simulink model "ProblemaTanques20240610"  (R2023b)
settings: Solver=ode4  StartTime=0.0  StopTime=100  FixedStep=.001  RelTol=1e-3
values from neighbouring files (symbols this model uses):
  Ts = 0.005    [Problema9_2024B.m]    (also in ScriptSimpleDiscretizacion20240617.m = 0.01)
libraries: cstblocks x3
settings Model: Creator=AlejandroGhersin  LastModifiedBy=AlejandroGhersin

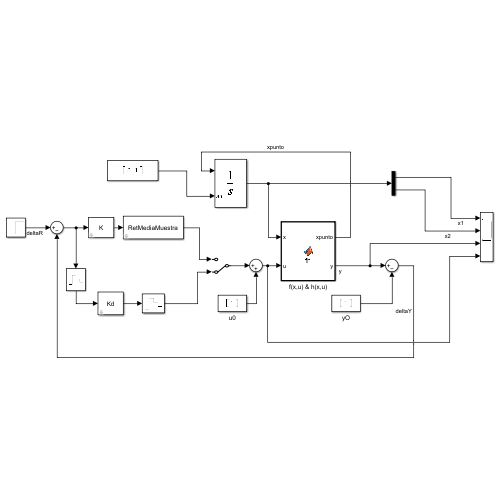
[thumbnail: Simulink's stored preview of the top-level diagram]
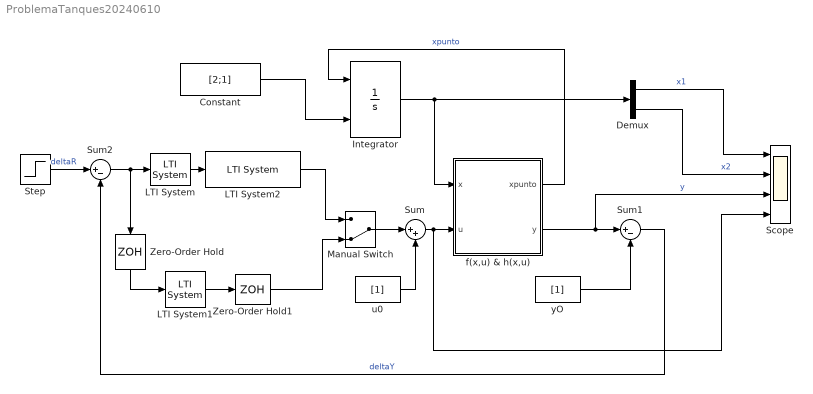
== system ProblemaTanques20240610 ==
  Constant : Constant  Value=[2;1]
  Demux : Demux  Outputs=2
  Integrator : Integrator  InitialConditionSource=external
  LTI System : cstblocks/LTI System  sys=K  IC=[]  PadeOrder=0
  LTI System1 : cstblocks/LTI System  sys=Kd  IC=[]  PadeOrder=0
  LTI System2 : cstblocks/LTI System  sys=RetMediaMuestra  IC=[]  PadeOrder=0
  Manual Switch : ManualSwitch  CurrentSetting=0
  Scope : Scope  NumInputPorts=4
  Step : Step  After=.2  SampleTime=0
  Sum : Sum  Inputs=|++
  Sum1 : Sum  Inputs=|+-
  Sum2 : Sum  Inputs=|+-
  Zero-Order Hold : ZeroOrderHold  SampleTime=Ts
  Zero-Order Hold1 : ZeroOrderHold  SampleTime=Ts
  f(x,u) & h(x,u) : MATLAB Function  TreatAsAtomicUnit=on
  u0 : Constant  Value=[1]
  yO : Constant  Value=[1]
  wires:
  Integrator/1 -> f(x,u) & h(x,u)/1(x), Demux/1
  Demux/2 -> Scope/2  "x2"
  f(x,u) & h(x,u)/1(xpunto) -> Integrator/1  "xpunto"
  Demux/1 -> Scope/1  "x1"
  Constant/1 -> Integrator/2
  u0/1 -> Sum/2
  Sum/1 -> Scope/4, f(x,u) & h(x,u)/2(u)
  f(x,u) & h(x,u)/2(y) -> Scope/3, Sum1/1  "y"
  yO/1 -> Sum1/2
  Sum2/1 -> LTI System/1, Zero-Order Hold/1
  Sum1/1 -> Sum2/2  "deltaY"
  Step/1 -> Sum2/1  "deltaR"
  Manual Switch/1 -> Sum/1
  LTI System/1 -> LTI System2/1
  LTI System1/1 -> Zero-Order Hold1/1
  Zero-Order Hold/1 -> LTI System1/1
  LTI System2/1 -> Manual Switch/1
  Zero-Order Hold1/1 -> Manual Switch/2

== matlab function ProblemaTanques20240610/f(x,u) & h(x,u) ==
  data: x input; xpunto output; u input; y output
function [xpunto,y] = fh(x,u)

% f(x,u);
xpunto1=u-sqrt(x(1)-x(2));
xpunto2=sqrt(x(1)-x(2)) - sqrt(x(2));

xpunto=[xpunto1;xpunto2];
% __________________
y = x(2); % h(x,u)
